simulink model "FormationSim"  (R2020b)
settings: Solver=ode45  StartTime=0.0  StopTime=15  FixedStep=0.01  MaxStep=0.01  RelTol=1e-3  EnableMultiTasking=on
values from neighbouring files (symbols this model uses):
  Adj_VL = [Adj connect; connect' 0]    [graph_create.m]
  Adj_VL_2 = [Adj_2 connect_2; connect_2' 0]    [graph_create.m]
  N = size(vehicle_pos.data,2)    [plot_animated_traj_2D.m]    (also in plot_animated_traj_3D.m)
undefined symbols (not defined in the file or in its folder): f_thrust_limit_up, g, k_aer_x, k_aer_y, k_aer_z, kd_ref, kdp, kdps, kdt, kdx, kdy, kdz, kp_ref, kpp, kpps, kpt, kpx, kpy, kpz, m, max_phi, max_theta, quad_physical, r_init, r_rel_1, r_rel_2, r_rel_3, xi_init
settings Model: Creator=Jens  LastModifiedBy=fcsou
settings DataIOCC: ReturnWorkspaceOutputs=off
settings OptimizationCC: LifeSpan=inf
settings DebuggingCC: SFUnexpectedBacktrackingDiag=warning  SFNoUnconditionalDefaultTransitionDiag=warning  ArithmeticOperatorsInVariantConditions=warning
settings SFSimCC: SimUseLocalCustomCode=off  CustomCodeUndefinedFunction=UseInterfaceOnly
settings RTWCC: RTWUseLocalCustomCode=off
settings CodeAppCC: StateflowObjectComments=on
settings GRTTargetCC: TargetLangStandard=C89/C90 (ANSI)
settings ConfigComp: CovMetricSettings=dw  CovSaveCumulativeToWorkspaceVar=on  CovSaveSingleToWorkspaceVar=on  CovExternalEMLEnable=off

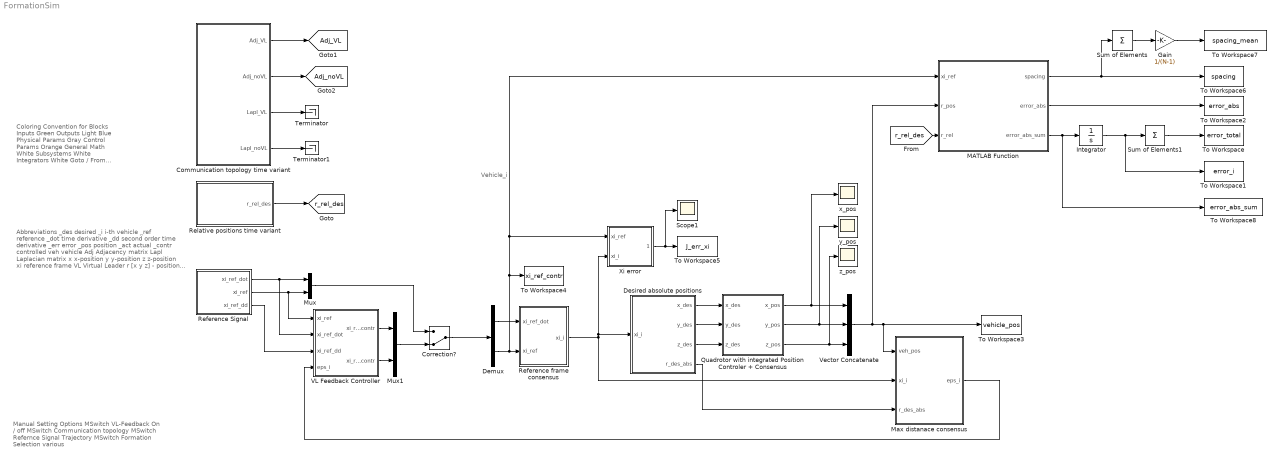
== system FormationSim ==
  note: Vehicle_i
  note: Manual Setting Options
      | MSwitch VL-Feedback On / off
      | MSwitch Communication topology
      | MSwitch Refernce Signal Trajectory
      | MSwitch Formation Selection various
  note: Abbreviations
      | _des desired
      | _i i-th vehicle
      | _ref reference
      | _dot time derivative
      | _dd second order time derivative
      | _err error
      | _pos position
      | _act actual
      | _contr controlled
      | veh vehicle
      | Adj Adjacency matrix
      | Lapl Laplacian matrix
      | x x-position
      | y y-position
      | z z-position
      | xi reference frame
      | VL Virtual Leader
      | r [x y z] - position
      | _rel relative in virtual frame
      | quad quadrotor
  note: Coloring Convention for Blocks
      | Inputs Green
      | Outputs Light Blue
      | Physical Params Gray
      | Control Params Orange
      | General Math White
      | Subsystems White
      | Integrators White
      | Goto / From Yellow
  Communication topology time variant : Subsystem
  Correction? : ManualSwitch  CurrentSetting=0
  Demux : Demux  Outputs=2
  Desired absolute positions : Subsystem
  Gain : Gain  Gain=1/(N-1)
  Integrator : Integrator
  MATLAB Function : MATLAB Function  TreatAsAtomicUnit=on
  Max distanace consensus : Subsystem
  Mux : Mux  Inputs=2
  Mux1 : Mux  Inputs=2
  Quadrotor with integrated Position Controler + Consensus : Subsystem
  Reference Signal : Subsystem
  Reference frame consensus : Subsystem
  Relative positions time variant : Subsystem
  Scope1 : Scope
  Sum of Elements : Sum  Inputs=+
  Sum of Elements1 : Sum  Inputs=+
  Terminator : Terminator
  Terminator1 : Terminator
  To Workspace : ToWorkspace  VariableName=error_total  SaveFormat=Timeseries  SampleTime=-1
  To Workspace1 : ToWorkspace  VariableName=error_i  SaveFormat=Timeseries  SampleTime=-1
  To Workspace2 : ToWorkspace  VariableName=error_abs  SaveFormat=Timeseries  SampleTime=-1
  To Workspace3 : ToWorkspace  VariableName=vehicle_pos  SaveFormat=Timeseries  SampleTime=-1
  To Workspace4 : ToWorkspace  VariableName=xi_ref_contr  SaveFormat=Timeseries  SampleTime=-1
  To Workspace5 : ToWorkspace  VariableName=J_err_xi  SaveFormat=Timeseries  SampleTime=-1
  To Workspace6 : ToWorkspace  VariableName=spacing  SaveFormat=Timeseries  SampleTime=-1
  To Workspace7 : ToWorkspace  VariableName=spacing_mean  SaveFormat=Timeseries  SampleTime=-1
  To Workspace8 : ToWorkspace  VariableName=error_abs_sum  SaveFormat=Timeseries  SampleTime=-1
  VL Feedback Controller : Subsystem
  Vector Concatenate : Concatenate  NumInputs=3  Mode=Multidimensional array
  Xi error : Subsystem
  x_pos : Scope
  y_pos : Scope
  z_pos : Scope
  tag scope: Adj_VL=global, Adj_noVL=global, r_rel_des=global
  wires:
  Communication topology time variant/1(Adj_VL) -> [Adj_VL]
  Reference Signal/2(xi_ref) -> VL Feedback Controller/1(xi_ref), Mux/2
  Reference Signal/1(xi_ref_dot) -> VL Feedback Controller/2(xi_ref_dot), Mux/1
  VL Feedback Controller/1(xi_ref_dot_contr) -> Mux1/1
  VL Feedback Controller/2(xi_ref_contr) -> Mux1/2
  Mux/1 -> Correction?/1
  Mux1/1 -> Correction?/2
  Correction?/1 -> Demux/1
  Relative positions time variant/1(r_rel_des) -> [r_rel_des]
  Quadrotor with integrated Position Controler + Consensus/3(z_pos) -> Vector Concatenate/3, z_pos/1
  Desired absolute positions/1(x_des) -> Quadrotor with integrated Position Controler + Consensus/1(x_des)
  Demux/1 -> Reference frame consensus/1(xi_ref_dot)
  Quadrotor with integrated Position Controler + Consensus/2(y_pos) -> Vector Concatenate/2, y_pos/1
  Desired absolute positions/3(z_des) -> Quadrotor with integrated Position Controler + Consensus/3(z_des)
  Quadrotor with integrated Position Controler + Consensus/1(x_pos) -> Vector Concatenate/1, x_pos/1
  Vector Concatenate/1 -> To Workspace3/1, Max distanace consensus/1(veh_pos), MATLAB Function/2(r_pos)
  Reference frame consensus/1(xi_i) -> Max distanace consensus/2(xi_i), Xi error/2(xi_i), Desired absolute positions/1(xi_i)
  Demux/2 -> To Workspace4/1, MATLAB Function/1(xi_ref), Xi error/1(xi_ref), Reference frame consensus/2(xi_ref)
  Desired absolute positions/2(y_des) -> Quadrotor with integrated Position Controler + Consensus/2(y_des)
  Max distanace consensus/1(eps_i) -> VL Feedback Controller/4(eps_i)
  [r_rel_des] -> MATLAB Function/3(r_rel)
  Communication topology time variant/2(Adj_noVL) -> [Adj_noVL]
  Communication topology time variant/3(Lapl_VL) -> Terminator/1
  Communication topology time variant/4(Lapl_noVL) -> Terminator1/1
  Integrator/1 -> Sum of Elements1/1, To Workspace1/1
  Reference Signal/3(xi_ref_dd) -> VL Feedback Controller/3(xi_ref_dd)
  Xi error/1("J_err_xi ") -> Scope1/1, To Workspace5/1
  Desired absolute positions/4(r_des_abs) -> Max distanace consensus/3(r_des_abs)
  Sum of Elements/1 -> Gain/1
  Gain/1 -> To Workspace7/1
  MATLAB Function/1(spacing) -> To Workspace6/1, Sum of Elements/1
  MATLAB Function/3(error_abs_sum) -> To Workspace8/1, Integrator/1
  Sum of Elements1/1 -> To Workspace/1
  MATLAB Function/2(error_abs) -> To Workspace2/1

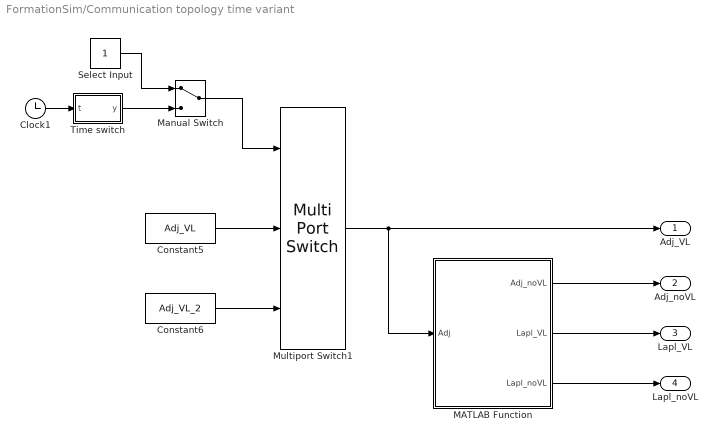
== system FormationSim/Communication topology time variant ==
  Clock1 : Clock
  Constant5 : Constant  Value=Adj_VL
  Constant6 : Constant  Value=Adj_VL_2
  MATLAB Function : MATLAB Function  TreatAsAtomicUnit=on
  Manual Switch : ManualSwitch
  Multiport Switch1 : MultiPortSwitch  Inputs=2
  Select Input : Constant
  Time switch : MATLAB Function  TreatAsAtomicUnit=on
  Adj_VL : Outport
  Adj_noVL : Outport  Port=2
  Lapl_VL : Outport  Port=3
  Lapl_noVL : Outport  Port=4
  wires:
  Manual Switch/1 -> Multiport Switch1/1
  Clock1/1 -> Time switch/1(t)
  Constant6/1 -> Multiport Switch1/3
  Constant5/1 -> Multiport Switch1/2
  Select Input/1 -> Manual Switch/1
  Time switch/1(y) -> Manual Switch/2
  Multiport Switch1/1 -> MATLAB Function/1(Adj), Adj_VL/1
  MATLAB Function/1(Adj_noVL) -> Adj_noVL/1
  MATLAB Function/2(Lapl_VL) -> Lapl_VL/1
  MATLAB Function/3(Lapl_noVL) -> Lapl_noVL/1

== system FormationSim/Desired absolute positions ==
  xi_i : Inport
  Desired absolute positions : MATLAB Function  TreatAsAtomicUnit=on
  To Workspace2 : ToWorkspace  VariableName=des_pos  SaveFormat=Timeseries  SampleTime=-1
  x_des : Outport
  y_des : Outport  Port=2
  z_des : Outport  Port=3
  r_des_abs : Outport  Port=4
  wires:
  Desired absolute positions/1(x_des) -> x_des/1
  Desired absolute positions/4(r_des) -> r_des_abs/1, To Workspace2/1
  Desired absolute positions/3(z_des) -> z_des/1
  Desired absolute positions/2(y_des) -> y_des/1
  xi_i/1 -> Desired absolute positions/1(xi_i)
  [r_rel_des] -> Desired absolute positions/2(r_relative)

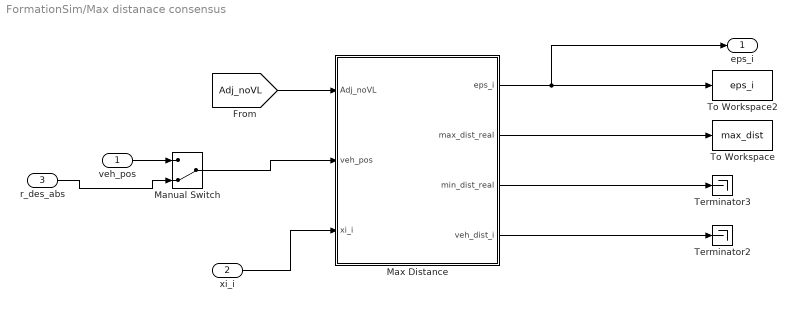
== system FormationSim/Max distanace consensus ==
  veh_pos : Inport
  xi_i : Inport  Port=2
  r_des_abs : Inport  Port=3
  Manual Switch : ManualSwitch  CurrentSetting=0
  Max Distance : MATLAB Function  TreatAsAtomicUnit=on
  Terminator2 : Terminator
  Terminator3 : Terminator
  To Workspace : ToWorkspace  VariableName=max_dist  SaveFormat=Timeseries  SampleTime=-1
  To Workspace2 : ToWorkspace  VariableName=eps_i  SaveFormat=Timeseries  SampleTime=-1
  eps_i : Outport
  wires:
  xi_i/1 -> Max Distance/3(xi_i)
  [Adj_noVL] -> Max Distance/1(Adj_noVL)
  Max Distance/1(eps_i) -> eps_i/1, To Workspace2/1
  Max Distance/2(max_dist_real) -> To Workspace/1
  Max Distance/4(veh_dist_i) -> Terminator2/1
  Max Distance/3(min_dist_real) -> Terminator3/1
  veh_pos/1 -> Manual Switch/1
  Manual Switch/1 -> Max Distance/2(veh_pos)
  r_des_abs/1 -> Manual Switch/2

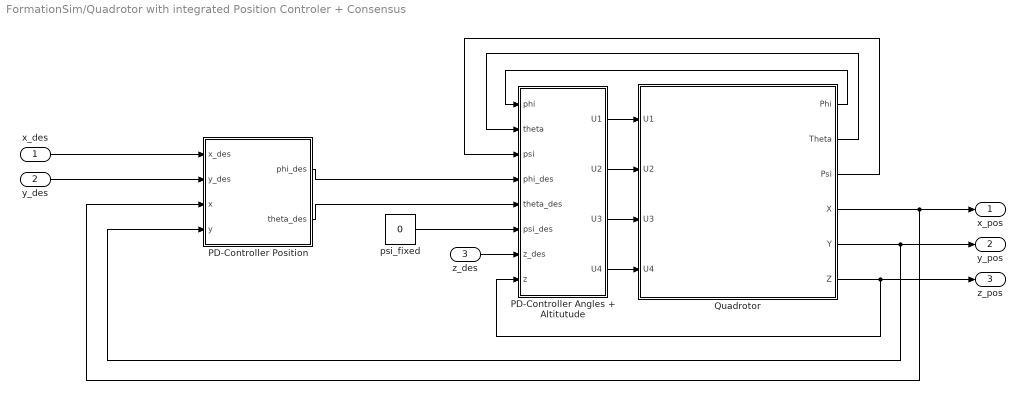
== system FormationSim/Quadrotor with integrated Position Controler + Consensus ==
  x_des : Inport
  y_des : Inport  Port=2
  z_des : Inport  Port=3
  PD-Controller Angles + Altitutude : Subsystem
  PD-Controller Position : Subsystem
  Quadrotor : Subsystem
  psi_fixed : Constant  Value=0
  x_pos : Outport
  y_pos : Outport  Port=2
  z_pos : Outport  Port=3
  wires:
  PD-Controller Angles + Altitutude/1(U1) -> Quadrotor/1(U1)
  Quadrotor/3(Psi) -> PD-Controller Angles + Altitutude/3(psi)
  Quadrotor/6(Z) -> PD-Controller Angles + Altitutude/8(z), z_pos/1
  PD-Controller Position/1(phi_des) -> PD-Controller Angles + Altitutude/4(phi_des)
  Quadrotor/2(Theta) -> PD-Controller Angles + Altitutude/2(theta)
  PD-Controller Position/2(theta_des) -> PD-Controller Angles + Altitutude/5(theta_des)
  z_des/1 -> PD-Controller Angles + Altitutude/7(z_des)
  Quadrotor/1(Phi) -> PD-Controller Angles + Altitutude/1(phi)
  PD-Controller Angles + Altitutude/3(U3) -> Quadrotor/3(U3)
  PD-Controller Angles + Altitutude/2(U2) -> Quadrotor/2(U2)
  PD-Controller Angles + Altitutude/4(U4) -> Quadrotor/4(U4)
  y_des/1 -> PD-Controller Position/2(y_des)
  x_des/1 -> PD-Controller Position/1(x_des)
  Quadrotor/4(X) -> PD-Controller Position/3(x), x_pos/1
  Quadrotor/5(Y) -> PD-Controller Position/4(y), y_pos/1
  psi_fixed/1 -> PD-Controller Angles + Altitutude/6(psi_des)

== system FormationSim/Reference Signal ==
  Integrator : Integrator  InitialCondition=[0;0;0;0;0;0]
  Integrator1 : Integrator
  Mux2 : Mux  Inputs=6
  Scope : Scope
  To Workspace : ToWorkspace  VariableName=xi_ref  SaveFormat=Timeseries  SampleTime=-1
  accelerations : Subsystem
  angular acclerations : Subsystem
  xi_ref_dot : Outport
  xi_ref : Outport  Port=2
  xi_ref_dd : Outport  Port=3
  wires:
  Mux2/1 -> xi_ref_dd/1, Integrator1/1
  Integrator/1 -> Scope/1, To Workspace/1, xi_ref/1
  accelerations/1(x_ref_dd) -> Mux2/1
  accelerations/2(y_ref_dd) -> Mux2/2
  accelerations/3(z_ref_dd) -> Mux2/3
  angular acclerations/1(alpha_ref_dd) -> Mux2/4
  angular acclerations/2(beta_ref_dd) -> Mux2/5
  angular acclerations/3(gamma_ref_dd) -> Mux2/6
  Integrator1/1 -> Integrator/1, xi_ref_dot/1

== system FormationSim/Reference frame consensus ==
  xi_ref_dot : Inport
  xi_ref : Inport  Port=2
  Consensus : MATLAB Function  TreatAsAtomicUnit=on
  Integrator : Integrator  InitialCondition=xi_init
  Memory : Memory
  To Workspace : ToWorkspace  VariableName=xi_i  SaveFormat=Timeseries  SampleTime=-1
  xi_i : Outport
  wires:
  [Adj_VL] -> Consensus/1(Adj_VL)
  xi_ref_dot/1 -> Consensus/2(xi_ref_dot)
  xi_ref/1 -> Consensus/3(xi_ref)
  Memory/1 -> Consensus/5(xi_i_dot)
  Consensus/1(u_xi_i) -> Integrator/1, Memory/1
  Integrator/1 -> xi_i/1, To Workspace/1, Consensus/4(xi_i)

== system FormationSim/Relative positions time variant ==
  Clock : Clock
  Formation 1 : Constant  Value=r_rel_1
  Formation 2 : Constant  Value=r_rel_2
  Formation 3 : Constant  Value=r_rel_3
  MSwitch1 : ManualSwitch
  Multiport Switch : MultiPortSwitch
  Static output selection : Constant  Value=3
  Time variable output selection : MATLAB Function  TreatAsAtomicUnit=on
  r_rel_des : Outport
  wires:
  Static output selection/1 -> MSwitch1/1
  Time variable output selection/1(y) -> MSwitch1/2
  MSwitch1/1 -> Multiport Switch/1
  Formation 1/1 -> Multiport Switch/2
  Formation 2/1 -> Multiport Switch/3
  Clock/1 -> Time variable output selection/1(t)
  Multiport Switch/1 -> r_rel_des/1
  Formation 3/1 -> Multiport Switch/4

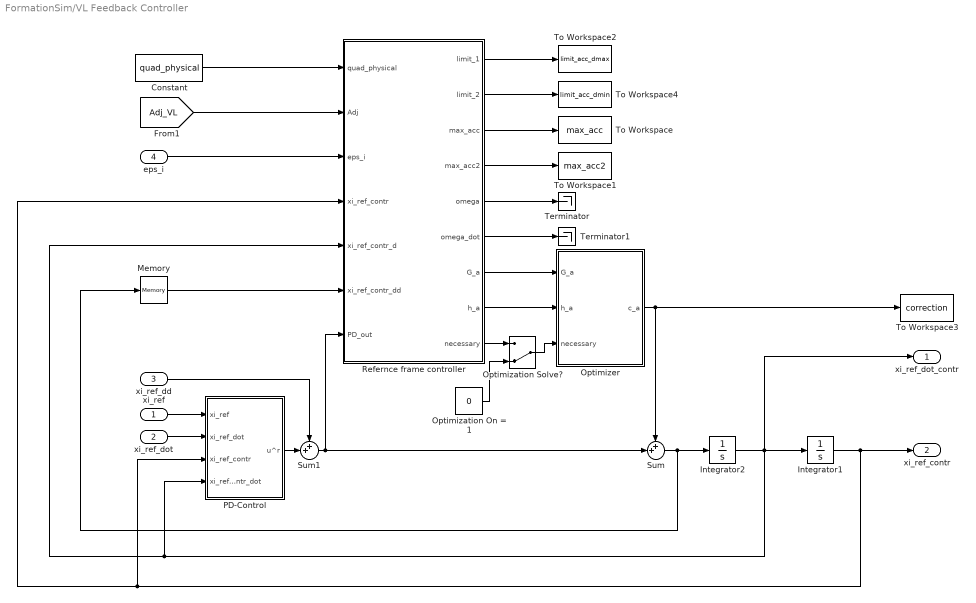
== system FormationSim/VL Feedback Controller ==
  xi_ref : Inport
  xi_ref_dot : Inport  Port=2
  xi_ref_dd : Inport  Port=3
  eps_i : Inport  Port=4
  Constant : Constant  Value=quad_physical
  Integrator1 : Integrator
  Integrator2 : Integrator
  Memory : Memory
  Optimization On = 1 : Constant  Value=0
  Optimization Solve? : ManualSwitch  CurrentSetting=0
  Optimizer : MATLAB Function  TreatAsAtomicUnit=on
  PD-Control : Subsystem
  Refernce frame controller : MATLAB Function  TreatAsAtomicUnit=on
  Sum : Sum  Inputs=++|
  Sum1 : Sum  Inputs=++|
  Terminator : Terminator
  Terminator1 : Terminator
  To Workspace : ToWorkspace  VariableName=max_acc  SaveFormat=Timeseries  SampleTime=-1
  To Workspace1 : ToWorkspace  VariableName=max_acc2  SaveFormat=Timeseries  SampleTime=-1
  To Workspace2 : ToWorkspace  VariableName=limit_acc_dmax  SaveFormat=Timeseries  SampleTime=-1
  To Workspace3 : ToWorkspace  VariableName=correction  SaveFormat=Timeseries  SampleTime=-1
  To Workspace4 : ToWorkspace  VariableName=limit_acc_dmin  SaveFormat=Timeseries  SampleTime=-1
  xi_ref_dot_contr : Outport
  xi_ref_contr : Outport  Port=2
  wires:
  [Adj_VL] -> Refernce frame controller/2(Adj)
  eps_i/1 -> Refernce frame controller/3(eps_i)
  Refernce frame controller/3(max_acc) -> To Workspace/1
  Refernce frame controller/4(max_acc2) -> To Workspace1/1
  xi_ref/1 -> PD-Control/1(xi_ref)
  Sum/1 -> Memory/1, Integrator2/1
  Refernce frame controller/5(omega) -> Terminator/1
  Refernce frame controller/6(omega_dot) -> Terminator1/1
  Refernce frame controller/7(G_a) -> Optimizer/1(G_a)
  Refernce frame controller/8(h_a) -> Optimizer/2(h_a)
  Optimizer/1(c_a) -> Sum/1, To Workspace3/1
  Memory/1 -> Refernce frame controller/6(xi_ref_contr_dd)
  Integrator2/1 -> xi_ref_dot_contr/1, Integrator1/1, Refernce frame controller/5(xi_ref_contr_d), PD-Control/4(xi_ref_contr_dot)
  Integrator1/1 -> Refernce frame controller/4(xi_ref_contr), PD-Control/3(xi_ref_contr), xi_ref_contr/1
  Constant/1 -> Refernce frame controller/1(quad_physical)
  Refernce frame controller/1(limit_1) -> To Workspace2/1
  Optimization On = 1/1 -> Optimization Solve?/2
  Refernce frame controller/9(necessary) -> Optimization Solve?/1
  Optimization Solve?/1 -> Optimizer/3(necessary)
  Refernce frame controller/2(limit_2) -> To Workspace4/1
  xi_ref_dot/1 -> PD-Control/2(xi_ref_dot)
  Sum1/1 -> Sum/2, Refernce frame controller/7(PD_out)
  PD-Control/1(u^r) -> Sum1/2
  xi_ref_dd/1 -> Sum1/1

== system FormationSim/Xi error ==
  xi_ref : Inport
  xi_i : Inport  Port=2
  Integrator : Integrator
  Integrator1 : Integrator
  Scope : Scope
  To Workspace : ToWorkspace  VariableName=J_xi_a  SaveFormat=Timeseries  SampleTime=-1
  Xi error : MATLAB Function  TreatAsAtomicUnit=on
  "J_err_xi " : Outport
  wires:
  Xi error/1(err_xi) -> Integrator/1
  Integrator/1 -> "J_err_xi "/1
  xi_ref/1 -> Xi error/1(xi_ref)
  xi_i/1 -> Xi error/2(xi_i)
  Xi error/2(err_xi_alpha) -> Integrator1/1
  Integrator1/1 -> Scope/1, To Workspace/1

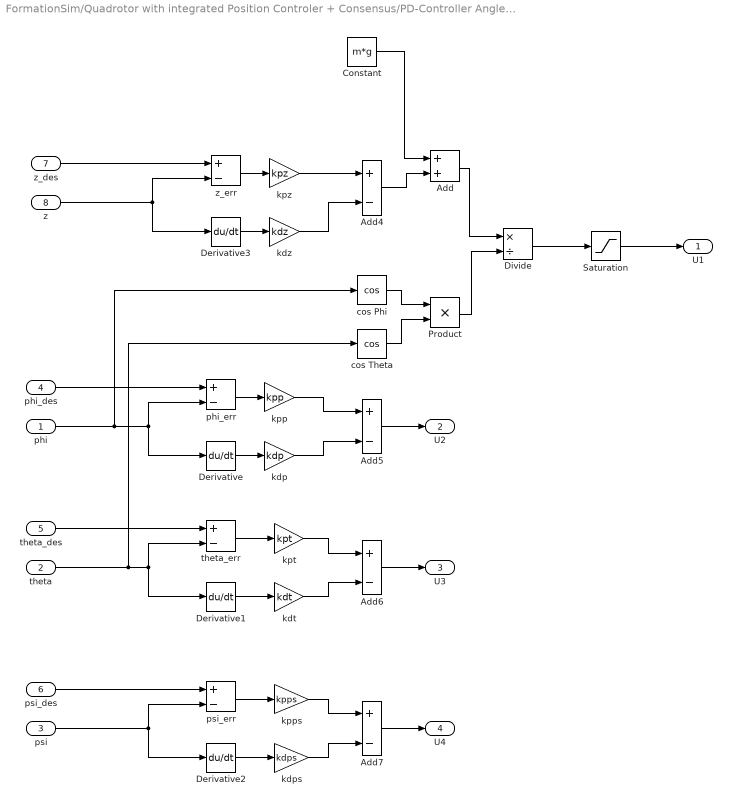
== system FormationSim/Quadrotor with integrated Position Controler + Consensus/PD-Controller Angles + Altitutude ==
  phi : Inport
  theta : Inport  Port=2
  psi : Inport  Port=3
  phi_des : Inport  Port=4
  theta_des : Inport  Port=5
  psi_des : Inport  Port=6
  z_des : Inport  Port=7
  z : Inport  Port=8
  Add : Sum
  Add{4..7} (4 alike) : Sum  Inputs=+-
  Constant : Constant  Value=m*g
  Derivative{,1..3} (4 alike) : Derivative
  Divide : Product  Inputs=*/
  Product : Product  RndMeth=Zero
  Saturation : Saturate  UpperLimit=f_thrust_limit_up  LowerLimit=0  ZeroCross=off
  cos Phi : Trigonometry  Operator=cos
  cos Theta : Trigonometry  Operator=cos
  kdp : Gain  Gain=kdp
  kdps : Gain  Gain=kdps
  kdt : Gain  Gain=kdt
  kdz : Gain  Gain=kdz
  kpp : Gain  Gain=kpp
  kpps : Gain  Gain=kpps
  kpt : Gain  Gain=kpt
  kpz : Gain  Gain=kpz
  phi_err : Sum  Inputs=+-
  psi_err : Sum  Inputs=+-
  theta_err : Sum  Inputs=+-
  z_err : Sum  Inputs=+-
  U1 : Outport
  U2 : Outport  Port=2
  U3 : Outport  Port=3
  U4 : Outport  Port=4
  wires:
  phi/1 -> Derivative/1, phi_err/2, cos Phi/1
  theta/1 -> Derivative1/1, theta_err/2, cos Theta/1
  psi/1 -> Derivative2/1, psi_err/2
  phi_des/1 -> phi_err/1
  theta_des/1 -> theta_err/1
  psi_des/1 -> psi_err/1
  phi_err/1 -> kpp/1
  Derivative/1 -> kdp/1
  theta_err/1 -> kpt/1
  Derivative1/1 -> kdt/1
  psi_err/1 -> kpps/1
  Derivative2/1 -> kdps/1
  z/1 -> Derivative3/1, z_err/2
  z_des/1 -> z_err/1
  z_err/1 -> kpz/1
  Derivative3/1 -> kdz/1
  kpz/1 -> Add4/1
  kdz/1 -> Add4/2
  kpp/1 -> Add5/1
  kdp/1 -> Add5/2
  Add5/1 -> U2/1
  kpt/1 -> Add6/1
  kdt/1 -> Add6/2
  Add6/1 -> U3/1
  kpps/1 -> Add7/1
  kdps/1 -> Add7/2
  Add7/1 -> U4/1
  cos Phi/1 -> Product/1
  cos Theta/1 -> Product/2
  Add4/1 -> Add/2
  Add/1 -> Divide/1
  Product/1 -> Divide/2
  Constant/1 -> Add/1
  Saturation/1 -> U1/1
  Divide/1 -> Saturation/1

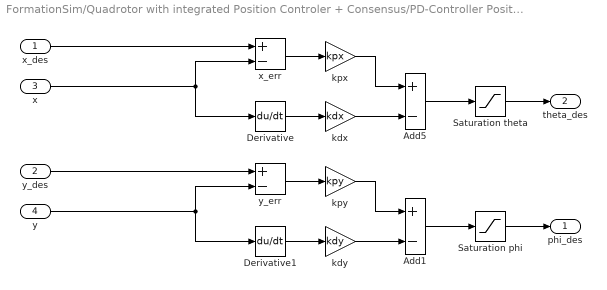
== system FormationSim/Quadrotor with integrated Position Controler + Consensus/PD-Controller Position ==
  x_des : Inport
  y_des : Inport  Port=2
  x : Inport  Port=3
  y : Inport  Port=4
  Add1 : Sum  Inputs=+-
  Add5 : Sum  Inputs=+-
  Derivative : Derivative
  Derivative1 : Derivative
  Saturation phi : Saturate  UpperLimit=max_phi  LowerLimit=-max_phi  ZeroCross=off
  Saturation theta : Saturate  UpperLimit=max_theta  LowerLimit=-max_theta  ZeroCross=off
  kdx : Gain  Gain=kdx
  kdy : Gain  Gain=kdy
  kpx : Gain  Gain=kpx
  kpy : Gain  Gain=kpy
  x_err : Sum  Inputs=+-
  y_err : Sum  Inputs=+-
  phi_des : Outport
  theta_des : Outport  Port=2
  wires:
  x/1 -> Derivative/1, x_err/2
  x_des/1 -> x_err/1
  x_err/1 -> kpx/1
  Derivative/1 -> kdx/1
  kpx/1 -> Add5/1
  kdx/1 -> Add5/2
  Add5/1 -> Saturation theta/1
  y/1 -> Derivative1/1, y_err/2
  y_err/1 -> kpy/1
  Derivative1/1 -> kdy/1
  kpy/1 -> Add1/1
  Add1/1 -> Saturation phi/1
  y_des/1 -> y_err/1
  Saturation theta/1 -> theta_des/1
  Saturation phi/1 -> phi_des/1
  kdy/1 -> Add1/2

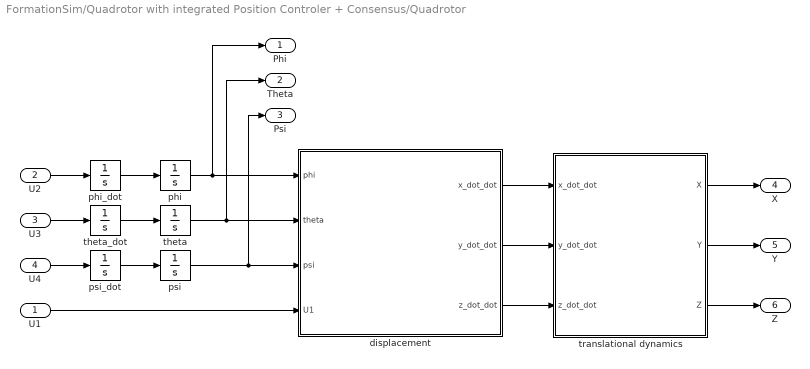
== system FormationSim/Quadrotor with integrated Position Controler + Consensus/Quadrotor ==
  U1 : Inport
  U2 : Inport  Port=2
  U3 : Inport  Port=3
  U4 : Inport  Port=4
  displacement : Subsystem
  phi : Integrator  ZeroCross=off
  phi_dot : Integrator
  psi : Integrator  ZeroCross=off
  psi_dot : Integrator  ZeroCross=off
  theta : Integrator  ZeroCross=off
  theta_dot : Integrator  ZeroCross=off
  translational dynamics : Subsystem
  Phi : Outport
  Theta : Outport  Port=2
  Psi : Outport  Port=3
  X : Outport  Port=4
  Y : Outport  Port=5
  Z : Outport  Port=6
  wires:
  U2/1 -> phi_dot/1
  U3/1 -> theta_dot/1
  U4/1 -> psi_dot/1
  phi_dot/1 -> phi/1
  theta_dot/1 -> theta/1
  psi_dot/1 -> psi/1
  phi/1 -> displacement/1(phi), Phi/1
  theta/1 -> displacement/2(theta), Theta/1
  psi/1 -> Psi/1, displacement/3(psi)
  U1/1 -> displacement/4(U1)
  displacement/1(x_dot_dot) -> translational dynamics/1(x_dot_dot)
  displacement/2(y_dot_dot) -> translational dynamics/2(y_dot_dot)
  displacement/3(z_dot_dot) -> translational dynamics/3(z_dot_dot)
  translational dynamics/1(X) -> X/1
  translational dynamics/2(Y) -> Y/1
  translational dynamics/3(Z) -> Z/1

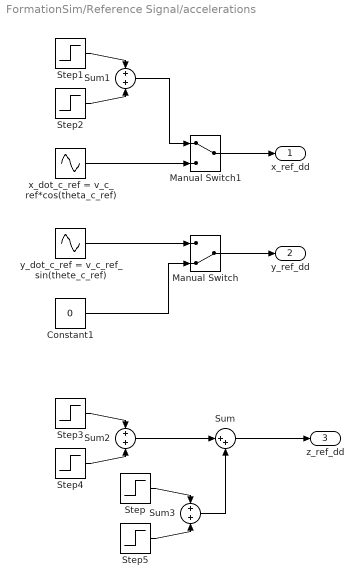
== system FormationSim/Reference Signal/accelerations ==
  Constant1 : Constant  Value=0
  Manual Switch : ManualSwitch  CurrentSetting=0
  Manual Switch1 : ManualSwitch
  Step : Step  Time=8  After=-1.3  SampleTime=0
  Step1 : Step  Time=0  After=0.4  SampleTime=0
  Step2 : Step  Time=2  After=-0.4  SampleTime=0
  Step3 : Step  Time=0  After=1.3  SampleTime=0
  Step4 : Step  Time=2  After=-1.3  SampleTime=0
  Step5 : Step  Time=10  After=1.3  SampleTime=0
  Sum : Sum  Inputs=|++
  Sum1 : Sum
  Sum2 : Sum
  Sum3 : Sum
  x_dot_c_ref = v_c_ref*cos(theta_c_ref) : Sin  Amplitude=9*pi/500  Frequency=pi/50  Phase=pi/2  SampleTime=0
  y_dot_c_ref = v_c_ref_sin(thete_c_ref) : Sin  Amplitude=9*pi/500  Frequency=pi/50  SampleTime=0
  x_ref_dd : Outport
  y_ref_dd : Outport  Port=2
  z_ref_dd : Outport  Port=3
  wires:
  Manual Switch/1 -> y_ref_dd/1
  y_dot_c_ref = v_c_ref_sin(thete_c_ref)/1 -> Manual Switch/1
  Constant1/1 -> Manual Switch/2
  x_dot_c_ref = v_c_ref*cos(theta_c_ref)/1 -> Manual Switch1/2
  Manual Switch1/1 -> x_ref_dd/1
  Sum1/1 -> Manual Switch1/1
  Sum/1 -> z_ref_dd/1
  Step2/1 -> Sum1/2
  Step1/1 -> Sum1/1
  Step4/1 -> Sum2/2
  Step3/1 -> Sum2/1
  Step5/1 -> Sum3/2
  Step/1 -> Sum3/1
  Sum3/1 -> Sum/2
  Sum2/1 -> Sum/1

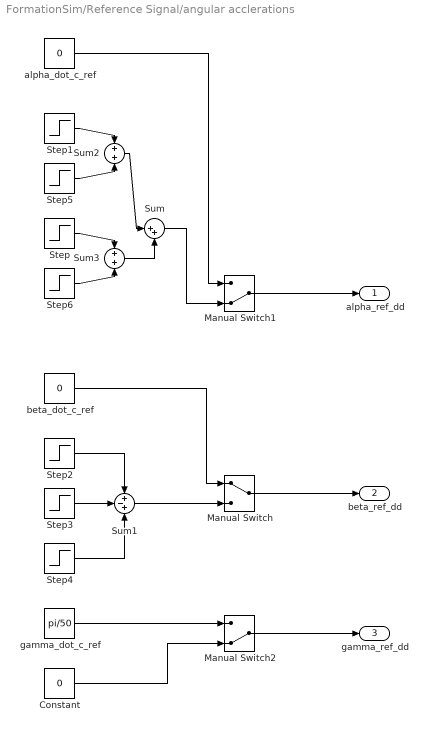
== system FormationSim/Reference Signal/angular acclerations ==
  Constant : Constant  Value=0
  Manual Switch : ManualSwitch
  Manual Switch1 : ManualSwitch  CurrentSetting=0
  Manual Switch2 : ManualSwitch  CurrentSetting=0
  Step : Step  Time=5  After=-pi/2  SampleTime=0
  Step1 : Step  Time=4  After=pi/2  SampleTime=0
  Step2 : Step  Time=10  After=pi/30  SampleTime=0
  Step3 : Step  Time=15  After=pi/30*2  SampleTime=0
  Step4 : Step  Time=20  After=pi/30  SampleTime=0
  Step5 : Step  Time=5  After=-pi/2  SampleTime=0
  Step6 : Step  Time=6  After=pi/2  SampleTime=0
  Sum : Sum  Inputs=|++
  Sum1 : Sum  Inputs=+-+
  Sum2 : Sum
  Sum3 : Sum
  alpha_dot_c_ref : Constant  Value=0
  beta_dot_c_ref : Constant  Value=0
  gamma_dot_c_ref : Constant  Value=pi/50
  alpha_ref_dd : Outport
  beta_ref_dd : Outport  Port=2
  gamma_ref_dd : Outport  Port=3
  wires:
  Step2/1 -> Sum1/1
  alpha_dot_c_ref/1 -> Manual Switch1/1
  Manual Switch/1 -> beta_ref_dd/1
  beta_dot_c_ref/1 -> Manual Switch/1
  Step3/1 -> Sum1/2
  Step4/1 -> Sum1/3
  Manual Switch1/1 -> alpha_ref_dd/1
  Sum1/1 -> Manual Switch/2
  Manual Switch2/1 -> gamma_ref_dd/1
  gamma_dot_c_ref/1 -> Manual Switch2/1
  Constant/1 -> Manual Switch2/2
  Sum/1 -> Manual Switch1/2
  Step5/1 -> Sum2/2
  Step1/1 -> Sum2/1
  Step6/1 -> Sum3/2
  Step/1 -> Sum3/1
  Sum3/1 -> Sum/2
  Sum2/1 -> Sum/1

== system FormationSim/VL Feedback Controller/PD-Control ==
  xi_ref : Inport
  xi_ref_dot : Inport  Port=2
  xi_ref_contr : Inport  Port=3
  xi_ref_contr_dot : Inport  Port=4
  Add6 : Sum
  kdt : Gain  Gain=kd_ref
  kpt : Gain  Gain=kp_ref
  xi_ref_dot_err : Sum  Inputs=+-
  xi_ref_err : Sum  Inputs=+-
  u^r : Outport
  wires:
  xi_ref_err/1 -> kpt/1
  xi_ref/1 -> xi_ref_err/1
  kdt/1 -> Add6/2
  Add6/1 -> u^r/1
  kpt/1 -> Add6/1
  xi_ref_contr/1 -> xi_ref_err/2
  xi_ref_dot/1 -> xi_ref_dot_err/1
  xi_ref_contr_dot/1 -> xi_ref_dot_err/2
  xi_ref_dot_err/1 -> kdt/1

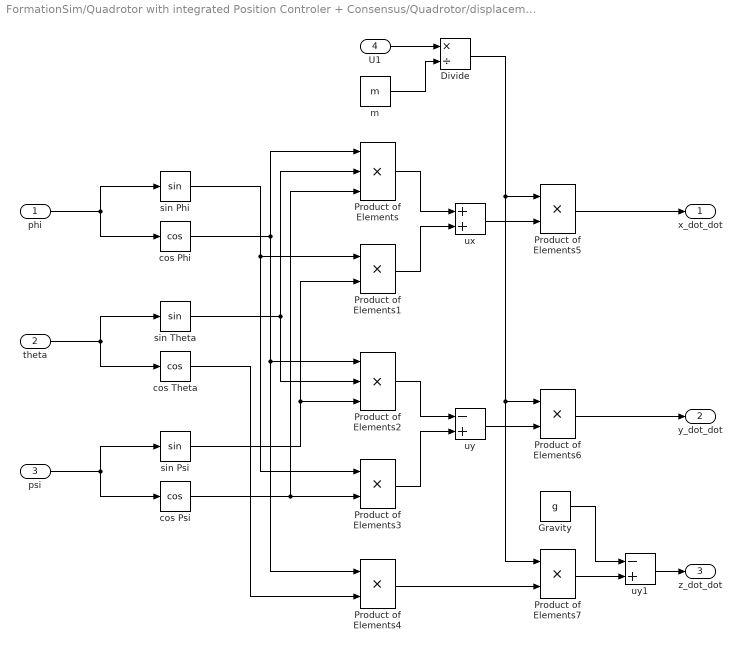
== system FormationSim/Quadrotor with integrated Position Controler + Consensus/Quadrotor/displacement ==
  phi : Inport
  theta : Inport  Port=2
  psi : Inport  Port=3
  U1 : Inport  Port=4
  Divide : Product  Inputs=*/
  Gravity : Constant  Value=g
  Product of Elements : Product  Inputs=3
  Product of Elements{1,3..7} (6 alike) : Product
  Product of Elements2 : Product  Inputs=3
  cos Phi : Trigonometry  Operator=cos
  cos Psi : Trigonometry  Operator=cos
  cos Theta : Trigonometry  Operator=cos
  m : Constant  Value=m
  sin Phi : Trigonometry
  sin Psi : Trigonometry
  sin Theta : Trigonometry
  ux : Sum
  uy : Sum  Inputs=-+
  uy1 : Sum  Inputs=-+
  x_dot_dot : Outport
  y_dot_dot : Outport  Port=2
  z_dot_dot : Outport  Port=3
  wires:
  phi/1 -> sin Phi/1, cos Phi/1
  theta/1 -> sin Theta/1, cos Theta/1
  psi/1 -> sin Psi/1, cos Psi/1
  sin Theta/1 -> Product of Elements/2, Product of Elements2/2
  cos Psi/1 -> Product of Elements/3, Product of Elements3/2
  cos Phi/1 -> Product of Elements/1, Product of Elements2/1, Product of Elements4/1
  sin Phi/1 -> Product of Elements1/1, Product of Elements3/1
  sin Psi/1 -> Product of Elements1/2, Product of Elements2/3
  Product of Elements/1 -> ux/1
  Product of Elements1/1 -> ux/2
  ux/1 -> Product of Elements5/2
  Product of Elements2/1 -> uy/1
  Product of Elements3/1 -> uy/2
  uy/1 -> Product of Elements6/2
  cos Theta/1 -> Product of Elements4/2
  Product of Elements4/1 -> Product of Elements7/2
  U1/1 -> Divide/1
  m/1 -> Divide/2
  Divide/1 -> Product of Elements5/1, Product of Elements6/1, Product of Elements7/1
  Product of Elements5/1 -> x_dot_dot/1
  Product of Elements6/1 -> y_dot_dot/1
  uy1/1 -> z_dot_dot/1
  Product of Elements7/1 -> uy1/2
  Gravity/1 -> uy1/1

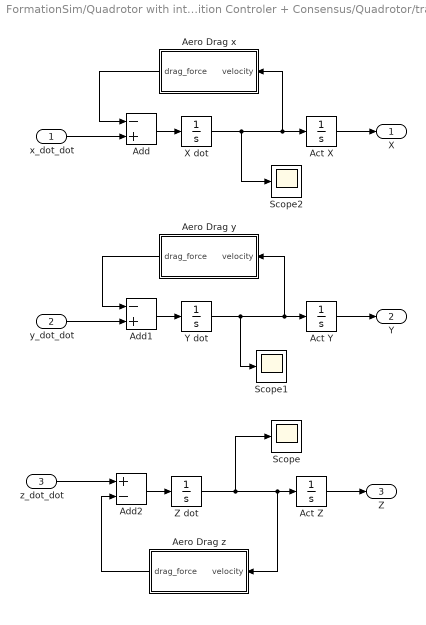
== system FormationSim/Quadrotor with integrated Position Controler + Consensus/Quadrotor/translational dynamics ==
  x_dot_dot : Inport
  y_dot_dot : Inport  Port=2
  z_dot_dot : Inport  Port=3
  Act X : Integrator  InitialCondition=r_init(1,:)
  Act Y : Integrator  InitialCondition=r_init(2,:)
  Act Z : Integrator  InitialCondition=r_init(3,:)
  Add : Sum  Inputs=-+
  Add1 : Sum  Inputs=-+
  Add2 : Sum  Inputs=+-
  Aero Drag x : Subsystem
  Aero Drag y : Subsystem
  Aero Drag z : Subsystem
  Scope : Scope
  Scope1 : Scope
  Scope2 : Scope
  X dot : Integrator
  Y dot : Integrator
  Z dot : Integrator
  X : Outport
  Y : Outport  Port=2
  Z : Outport  Port=3
  wires:
  Add1/1 -> Y dot/1
  Act Z/1 -> Z/1
  X dot/1 -> Scope2/1, Act X/1, Aero Drag x/1(velocity)
  Act Y/1 -> Y/1
  Aero Drag x/1(drag_force) -> Add/1
  y_dot_dot/1 -> Add1/2
  Y dot/1 -> Scope1/1, Aero Drag y/1(velocity), Act Y/1
  Aero Drag z/1(drag_force) -> Add2/2
  x_dot_dot/1 -> Add/2
  Aero Drag y/1(drag_force) -> Add1/1
  Z dot/1 -> Scope/1, Aero Drag z/1(velocity), Act Z/1
  Act X/1 -> X/1
  Add2/1 -> Z dot/1
  Add/1 -> X dot/1
  z_dot_dot/1 -> Add2/1

== system FormationSim/Quadrotor with integrated Position Controler + Consensus/Quadrotor/translational dynamics/Aero Drag x ==
  velocity : Inport
  Abs : Abs
  Gain : Gain  Gain=k_aer_x/m
  Product : Product
  drag_force : Outport
  wires:
  Product/1 -> Gain/1
  velocity/1 -> Product/1, Abs/1
  Gain/1 -> drag_force/1
  Abs/1 -> Product/2

== system FormationSim/Quadrotor with integrated Position Controler + Consensus/Quadrotor/translational dynamics/Aero Drag y ==
  velocity : Inport
  Abs : Abs
  Gain : Gain  Gain=k_aer_y/m
  Product : Product
  drag_force : Outport
  wires:
  Product/1 -> Gain/1
  velocity/1 -> Product/1, Abs/1
  Gain/1 -> drag_force/1
  Abs/1 -> Product/2

== system FormationSim/Quadrotor with integrated Position Controler + Consensus/Quadrotor/translational dynamics/Aero Drag z ==
  velocity : Inport
  Abs : Abs
  Gain : Gain  Gain=k_aer_z/m
  Product : Product
  drag_force : Outport
  wires:
  Product/1 -> Gain/1
  velocity/1 -> Product/1, Abs/1
  Gain/1 -> drag_force/1
  Abs/1 -> Product/2

== matlab function FormationSim/Communication topology time variant/MATLAB Function ==
  data: Adj input; Adj_noVL output; Lapl_VL output; Lapl_noVL output
function [Adj_noVL, Lapl_VL, Lapl_noVL] = lapl_adj_options(Adj)
%gives adjacency and laplacian matrix of graph with and without VL

% number of vehicles
N = size(Adj,1)-1;

% takes away last row and column
Adj_noVL = Adj(1:N,1:N);

% laplacian calculation after thesis definition
Lapl_VL = zeros(size(Adj));

for i=1:1:N+1
    for j=1:1:N+1
        if (i == j)
            % sets l(i,j) to the sum of the row without the diagonal
            % element
            Lapl_VL(i,j) = sum(Adj(i,:))-Adj(i,j);
        else
            Lapl_VL(i,j) = -Adj(i,j);
        end
    end
end
Lapl_noVL = Lapl_VL(1:N,1:N);

== matlab function FormationSim/VL Feedback Controller/Optimizer ==
  data: G_a input; c_a output; h_a input; necessary input
function c_a = correction(G_a,h_a,necessary)
% CORRECTION solves a QP problem to minimize c_a^T*H*c_a subjec to G_a*c_a
% < h_a. The solver is only active if indicated by the boolean necessary.
%
% Input:
%       G_a       - left side matrix of QP constraint
%       h_a       - right hand side vector of QP constraint
%       necessary - boolean which indicates if optimization necessary
% Ooutput:
%       c_a       - correction vector which solves optimization problem

c_a = zeros(6,1);
coder.extrinsic('quadprog')
if (necessary)
    H = diag([0.1;0.1;0.1;1;1;1]); % weight matrix H
    c_a = quadprog(H,zeros(6,1),G_a,h_a);
end

== matlab function FormationSim/MATLAB Function ==
  data: spacing output; xi_ref input; error_abs output; r_pos input; r_rel input; error_abs_sum output
function [spacing,error_abs,error_abs_sum] = err_calc(xi_ref, r_pos, r_rel)
%ERR_CALC calculates the squared error between the given reference frame
%xi_ref and each vehicle actual position.
%
% Input:
%     xi_ref       - virtual reference frame
%     r_pos        - position vector of vehicles
%     r_rel        - relative positions of vehicles in formation
% Output:
%     err_total    - total squared errror over all vehicles
%     err_i        - individual error per vehicle
%     err_coord    - error per coordinate axis
%     

% number of vehicles
N = size(r_pos,2);

% calculate desired absolute positions based on xi_ref
r_des_abs = zeros(size(r_pos));

phi = xi_ref(4);
theta = xi_ref(5);
psi = xi_ref(6);

% rotational matrix Rz
Dz = [cos(psi) -sin(psi) 0
    sin(psi)  cos(psi) 0
    0   0    1];

% rotational matrix Ry
Dy = [cos(theta)  0   sin(theta)
    0      1      0
    -sin(theta)  0   cos(theta)];

% rotational matrix Rx
Dx = [1     0         0
    0  cos(phi) -sin(phi)
    0  sin(phi)  cos(phi)];

%loop over each vehicle
for i=1:1:N     
    r_des_abs(:,i) = xi_ref(1:3) + Dz*Dy*Dx*r_rel(:,i);    
end

error = r_pos - r_des_abs;
error_abs = abs(error); 
error_abs_sum = sum(error_abs(2:3,:),1);
%squared error

%distance between vehicles
veh_spacing = sqrt(sum(diff(r_pos').^2,2));
veh_spacing_should = ones(N-1,1)*0.8;

spacing = abs(veh_spacing);

== matlab function FormationSim/Communication topology time variant/Time switch ==
  data: t input; y output
function y = time_switch(t)
%TIME_SWITCH gives time varying output for multiport switch
% Input:
%       t   - time
% Ooutput:
%       y   - multiport switch value
if (t >= 20 && t < 60)
    y = 2;
else
    y = 1;
end

== matlab function FormationSim/Reference frame consensus/Consensus ==
  data: Adj_VL input; u_xi_i output; xi_ref_dot input; xi_ref input; xi_i input; xi_i_dot input
function u_xi_i = consensus_xi(Adj_VL, xi_ref_dot, xi_ref, xi_i, xi_i_dot)
%CONSENSUS_XI calculates u_xi = xi_i_dot for all vehicles according to the consensus
%formula for time-varying reference state (access to the leader only to a subgroup)
% Inputs:
%       Adj_VL      - adjacency matrix
%       xi_ref_dot  - time derivative of the reference xi
%       xi_ref      - reference xi
%       xi_i        - vehicle i own understanding of reference frame
%       xi_i_dot    - vehicles i own understanding of the time derivative of xi
% Outputs:
%       u_xi_i       - control input of the i-th reference frame

% Number of vehicles
N = size(Adj_VL,1)-1;
% initialize output u_xi to zero
u_xi_i = zeros(6,N);

% scalar to influence convergence speed
gamma = 1;

% formula to calculate xi_dot_i = u_i for each vehicle compare to thesis
% u consists of six states per vehicle in a 6xN matrix / updates each
% vehicle after another (6 states per iteration of outer for loop)
for i=1:1:N
    eta = sum(Adj_VL(i,:));
    % if vehicle has no incoming connection (equal to eta = 0) u is set to zero therefore the
    % information states don't change and remain constant
    if (eta == 0)
        u_xi_i(:,i) = zeros(6,1);
    else
        temp = zeros(6,1);
        for j=1:1:N
            temp = temp + Adj_VL(i,j)*(xi_i_dot(:,j)-gamma*(xi_i(:,i)-xi_i(:,j)));
        end
        u_xi_i(:,i) = 1/eta * temp + 1/eta * Adj_VL(i,N+1)*(xi_ref_dot-gamma*(xi_i(:,i)-xi_ref));
    end    
end

== matlab function FormationSim/Relative positions time variant/Time variable output selection ==
  data: t input; y output
function y = time_switch(t)
%TIME_SWITCH gives time varying output for multiport switch
% Input:
%       t   - time
% Ooutput:
%       y   - multiport switch value
if (t < 5)
    y = 1;
elseif (t >= 5 && t < 12)
    y = 2;
elseif (t >= 50 && t < 100)
    y = 3;
else
    y = 1;
end

== matlab function FormationSim/Desired absolute positions/Desired absolute positions ==
  data: xi_i input; x_des output; r_relative input; y_des output; z_des output; r_des output
function [x_des,y_des,z_des,r_des]  = desired_pos_abs(xi_i, r_relative)
%DESIRED_POS_ABS computes the desired absolute positions depending on the
%reference frame of the vehicle and the relative coordinates of the desired
%formation (three dimensional coordinate transformation)
%
% Inputs:
%       xi_i    - reference frame of the i-th vehicle
%       r_relative  - vehicle formation shape in the reference frame
% Outputs:
%       x_des       - desired x-position of the vehicle
%       y_des       - desired y-position of the vehicle
%       z_des       - desired z-position of the vehicle
%       r_relative  - combination of x,y,z-position in a matrix for all veh

% set matrix nxn
r_des = zeros(size(r_relative));

%loop over each vehicle
for i=1:1:size(r_relative,2)
    
    % information state of the vehicle angle
    gamma = xi_i(6,i);
    beta = xi_i(5,i);
    alpha = xi_i(4,i);
    
    % rotational matrix Rz
    Dz = [cos(gamma) -sin(gamma) 0
        sin(gamma)  cos(gamma) 0
        0   0    1];
    
    % rotational matrix Ry
    Dy = [cos(beta)  0   sin(beta)
        0      1      0
        -sin(beta)  0   cos(beta)];
    
    % rotational matrix Rx
    Dx = [1     0         0
        0  cos(alpha) -sin(alpha)
        0  sin(alpha)  cos(alpha)];
     
    r_des(:,i) = xi_i(1:3,i) + Dz*Dy*Dx*r_relative(:,i);
end

x_des = r_des(1,:);
y_des = r_des(2,:);
z_des = r_des(3,:);

end

== matlab function FormationSim/Max distanace consensus/Max Distance ==
  data: Adj_noVL input; eps_i output; veh_pos input; xi_i input; max_dist_real output; min_dist_real output; veh_dist_i output
function [eps_i, max_dist_real, min_dist_real, veh_dist_i] = max_distance(Adj_noVL, veh_pos, xi_i)
%MAX_DISTANCE computes a maximum consensus of the distance from virtual
%center in the network. Using a synchronous broadcast algorithm were each
%sensor wakes up after a time and broadcasts his value to the other nodes.
%
% Inputs:
%   Ajd_noVl    - Ajacency without the VL
%   veh_pos     - current vehicles position in a 3xN matrix
%   xi_i        - state xi (virtual reference frame) of i-th vehicle
%
% Outputs:
%   max_dist_real   - real maximum distance in the whole network
%   min_dist_real   - real minimum distance in the whole network
%   veh_dist_i      - i-th vehicles distance from virtual center
%   eps_i           - state epsilon (max and min distance) of i-th vehicle


N = size(Adj_noVL,1);

veh_dist_i = veh_pos - xi_i(1:3,:);
max_dist_real = max(veh_dist_i,[],2);
min_dist_real = min(veh_dist_i,[],2);

eps_i = [veh_dist_i; veh_dist_i];

% loop over each vehicle five times to ensure convergence
for k=1:1:5
    for i=1:1:N
        for j=1:1:N
            if (Adj_noVL(i,j) == 1)
                % binary vector p to set only greater / smaller values
                p = [(eps_i(1:3,i) < eps_i(1:3,j));
                    (eps_i(4:6,i) > eps_i(4:6,j))];
                eps_i(:,i) = eps_i(:,j).*p + eps_i(:,i).*not(p);
            end 
        end
    end
end

== matlab function FormationSim/Xi error/Xi error ==
  data: xi_ref input; err_xi output; xi_i input; err_xi_alpha output
function [err_xi, err_xi_alpha] = err_ref(xi_ref, xi_i)
%ERR_REF computes the error between the vehicles information state and
%reference information.
% 
% Input:
%       - xi_ref    reference information state
%       - xi_i      vehicle information state
% Output:
%       - err_xi    absolute xi error

err_xi = abs(xi_ref*ones(1,size(xi_i,2)) - xi_i);
err_xi_alpha = err_xi(4,:);

== matlab function FormationSim/VL Feedback Controller/Refernce frame controller ==
  data: limit_1 output; limit_2 output; quad_physical input; max_acc output; max_acc2 output; Adj input; eps_i input; xi_ref_contr input; xi_ref_contr_d input; xi_ref_contr_dd input; omega output; omega_dot output; G_a output; h_a output; PD_out input; necessary output
function [limit_1, limit_2, max_acc, max_acc2, omega, omega_dot, G_a, h_a, necessary]  = xi_ref_contr(quad_physical ,Adj, eps_i, xi_ref_contr, xi_ref_contr_d, xi_ref_contr_dd, PD_out)
%XI_REF_CONTR is the controller for the reference frame xi depending on the
%the maximum distance of a reference trajectory computing the necessary
%values for the optimization (QP) problem.
%
% Inputs:
%       quad_physical   - physical constants of quadrotor
%       Adj             - adjacency matrix
%       eps_i           - maximum / minimum distance information state
%       xi_ref_contr    - controlled reference state
%       xi_ref_contr_d  - time derivitive of the reference state
%       xi_ref_contr_dd - second order time derivitive of reference state
%       PD_out          - Output of the PD-Controller for the reference
% Outputs:
%       limit_1         - current acceleration limit regarding d_max
%       limit_2         - current acceleration limit regarding d_min
%       max_acc         - current max required acceleration regarding d_max
%       min_acc2        - current max required acceleration regarding d_min
%       omega           - angular velocity of the reference frame in the
%                         inertial frame
%       omega_dot       - derivative of omega
%       G_a             - Matrix for inequality constraint optimization
%       h_a             - vector for ineqaulity constraint optimization
%       necessary       - boolean which activates the optimization
%                         algorithm if boundaries are hurt

%Quadrotor physical
% quad_physical = [m g k_aer_z k_aer_x k_aer_y f_thrust_limit_up max_theta max_phi];
m = quad_physical(1);
g = quad_physical(2);
k_aer_z = quad_physical(3);
k_aer_x = quad_physical(4);
k_aer_y = quad_physical(5);
f_thrust_limit_up = quad_physical(6);
theta_max = quad_physical(7);
phi_max = quad_physical(8);


% setup
N = size(Adj,1)-1; % number of vehicles
max_dist = zeros(3,1);
max_dist2 = zeros(3,1);

% information of maximal distance from connected vehicles to VL
flag = true;
for i=1:1:N
    if (Adj(N+1,i)==1)
        if (flag)
            max_dist = eps_i(1:3,i);
            max_dist2 = eps_i(4:6,i);
            flag = false;
        else
            % if multiple information available update only higher values
            max_dist = (eps_i(1:3,i) > max_dist).*eps_i(1:3,i) + not(eps_i(1:3,i) > max_dist).*eps_i(1:3,i);
            max_dist2 = (eps_i(4:6,i) < max_dist2).*eps_i(4:6,i) + not(eps_i(4:6,i) < max_dist2).*eps_i(4:6,i);
        end
    end
end

d1 = max_dist(1);
d2 = max_dist(2);
d3 = max_dist(3);
d4 = max_dist2(1);
d5 = max_dist2(2);
d6 = max_dist2(3);

% coordinate transformation of velocities and accelerations to inertial
% frame
alpha = xi_ref_contr(4); % euler angles
beta = xi_ref_contr(5);
gamma = xi_ref_contr(6);

alpha_dot = xi_ref_contr_d(4); % euler angles velocity
beta_dot = xi_ref_contr_d(5);
gamma_dot = xi_ref_contr_d(6);
delta_dot = [alpha_dot; beta_dot; gamma_dot];

alpha_dd = xi_ref_contr_dd(4); % angular accelerations
beta_dd = xi_ref_contr_dd(5);
gamma_dd = xi_ref_contr_dd(6);
delta_dd = [alpha_dd; beta_dd; gamma_dd];

v_center = xi_ref_contr_d(1:3); % center velocity of moving frame
a_center = xi_ref_contr_dd(1:3); % center accleration of moving frame

% rotation matrix from euler angles to inertial frame
rot = [ cos(gamma)*cos(beta) -sin(gamma)    0
        sin(gamma)*cos(beta)  cos(gamma)    0
       -sin(beta)              0        1];
   
rot_dot = [-gamma_dot*sin(gamma)*cos(beta)-beta_dot*cos(gamma)*sin(beta) -gamma_dot*cos(gamma) 0;
            gamma_dot*cos(gamma)*cos(beta)-beta_dot*sin(gamma)*sin(beta) -gamma_dot*sin(gamma) 0;
           -beta_dot*cos(beta) 0 0];

omega = rot*delta_dot; % angular velocities in inertial frame        
omega_dot = rot*delta_dd + rot_dot*delta_dot;

% expected current maximal velocity of most distant vehicles
max_veloc = v_center + cross(omega,max_dist);
max_veloc2 = v_center + cross(omega,max_dist2);

x_dot = max_veloc(1);
y_dot = max_veloc(2);
z_dot = max_veloc(3);

x_dot_2 = max_veloc2(1);
y_dot_2 = max_veloc2(2);
z_dot_2 = max_veloc2(3);
        
% expected current maximal acceleration of most distant vehicles
max_acc = a_center + cross(omega_dot,max_dist) + cross(omega,cross(omega,max_dist));
max_acc2 = a_center + cross(omega_dot,max_dist2) + cross(omega,cross(omega,max_dist2));

%Quad1_max zulässige Accelerations berechnen
drag_x = - k_aer_x*abs(x_dot)*x_dot/m;
drag_y = - k_aer_y*abs(y_dot)*y_dot/m;
drag_z = - k_aer_z*abs(z_dot)*z_dot/m;

drag_x_2 = - k_aer_x*abs(x_dot_2)*x_dot_2/m;
drag_y_2 = - k_aer_y*abs(y_dot_2)*y_dot_2/m;
drag_z_2 = - k_aer_z*abs(z_dot_2)*z_dot_2/m;

a_quad_plus_x = g*tan(theta_max) + drag_x;
a_quad_plus_y = -g*tan(-phi_max)/cos(theta_max) + drag_y;
a_quad_plus_z = f_thrust_limit_up/m - g + drag_z;

a_quad_plus_x_2 = g*tan(theta_max) + drag_x_2;
a_quad_plus_y_2 = -g*tan(-phi_max)/cos(theta_max) + drag_y_2;
a_quad_plus_z_2 = f_thrust_limit_up/m - g + drag_z_2;

a_quad_minus_x = -g*tan(theta_max) + drag_x;
a_quad_minus_y = -g*tan(phi_max)/cos(theta_max) + drag_y;
a_quad_minus_z = -g + drag_z;

a_quad_minus_x_2 = -g*tan(theta_max) + drag_x_2;
a_quad_minus_y_2 = -g*tan(phi_max)/cos(theta_max) + drag_y_2;
a_quad_minus_z_2 = -g + drag_z_2;

a_quad_plus = [a_quad_plus_x; a_quad_plus_y; a_quad_plus_z];
a_quad_minus = [a_quad_minus_x; a_quad_minus_y; a_quad_minus_z];

a_quad_plus_2 = [a_quad_plus_x_2; a_quad_plus_y_2; a_quad_plus_z_2];
a_quad_minus_2 = [a_quad_minus_x_2; a_quad_minus_y_2; a_quad_minus_z_2];

limit_1 = [a_quad_plus; a_quad_minus];
limit_2 = [a_quad_plus_2; a_quad_minus_2];

% check if optimization is necessary
temp = (max_acc > (a_quad_plus-[0.1;0.1;0.1]));
temp2 = (max_acc < (a_quad_minus+[0.1;0.1;0.1]));
temp3 = (max_acc2 > (a_quad_plus_2-[0.1;0.1;0.1]));
temp4 = (max_acc2 < (a_quad_minus_2+[0.1;0.1;0.1]));
% boolean == true if limits hit with extra margin of 0.1 because otherwise on/off switching of optimization
necessary = any([temp;temp2;temp3;temp4]); 

% calculating the matrix for inequaltiy constraint G_a*c_a < h_a for
% optimization
G_1 = [d3*cos(beta)*sin(gamma)+d2*sin(beta) cos(gamma)*d3 -d2;
    -d1*sin(beta)-d3*cos(beta)*cos(gamma) d3*sin(gamma) d1;
    d2*cos(beta)*cos(gamma)-d1*cos(beta)*sin(gamma) -d2*sin(gamma)-d1*cos(gamma) 0];

G_2 = [d6*cos(beta)*sin(gamma)+d5*sin(beta) cos(gamma)*d6 -d5;
    -d4*sin(beta)-d6*cos(beta)*cos(gamma) d6*sin(gamma) d4;
    d5*cos(beta)*cos(gamma)-d4*cos(beta)*sin(gamma) -d5*sin(gamma)-d4*cos(gamma) 0];

G_tilde_1 = [eye(3) G_1];
G_tilde_2 = [eye(3) G_2];

h_1 = cross(rot_dot*delta_dot, max_dist);
h_2 = cross(rot_dot*delta_dot, max_dist2);

h_tilde_1 = - cross(omega,cross(omega,max_dist)) - h_1 - G_tilde_1*PD_out;
h_tilde_2 = - cross(omega,cross(omega,max_dist2)) - h_2 - G_tilde_2*PD_out;

h_a = [a_quad_plus + h_tilde_1;
       -a_quad_minus - h_tilde_1;
       a_quad_plus_2 + h_tilde_2;
       -a_quad_minus_2 - h_tilde_2];

G_a = [G_tilde_1; -G_tilde_1; G_tilde_2; -G_tilde_2];
